simulink model "Drone_BBall_Friendly"  (R2020a)
settings: Solver=FixedStepAuto  StartTime=0.0  StopTime=60  FixedStep=.001  RelTol=1e-3
values from neighbouring files (symbols this model uses):
  b = .25*m    (= 0.25)    [Run_Match.m]
  b_ball = .02*m_ball    (= 0.01)    [Run_Match.m]
  b_F_hook = 100    [Run_Match.m]
  b_F_hoop = m_ball * 50    (= 25)    [Run_Match.m]
  b_F_R = m * 20    (= 20)    [Run_Match.m]
  b_F_R_ball = m_ball * 10    (= 5)    [Run_Match.m]
  b_F_R_hook = m_hook * 100    (= 10)    [Run_Match.m]
  B_hook = r_hook^2*6*m_ball*g    (= 0.2943)    [Run_Match.m]
  b_hook = 0.05*m_hook    (= 0.005)    [Run_Match.m]
  b_tether = 1    [Run_Match.m]
  b_th = .1*J    (= 0.0192708333333)    [Run_Match.m]
  b_th_ball = .05*J_ball    (= 0.0009)    [Run_Match.m]
  b_x_net = 80*m_ball*g    (= 392.4)    [Run_Match.m]
  b_y_net = .4*m_ball*g    (= 1.962)    [Run_Match.m]
  drone = struct([])    [Run_Match.m]    (also in animate_drone_bball.m = [-r+w -r-w -r -r r r r+w r-w;             h    h  h  0 0 h  )
  g = 9.81    [Run_Match.m]
  J = 1/4*m*r^2 + 1/12*m*(2*(r+r_M_R))^2    (= 0.192708333333)    [Run_Match.m]
  J_ball = 2/5*m_ball*r_ball^2    (= 0.018)    [Run_Match.m]
  k_f = 4    [Run_Match.m]
  k_F_hook = 10000    [Run_Match.m]
  k_F_hoop = m_ball * 5000    (= 2500)    [Run_Match.m]
  k_F_R = m * 10000    (= 10000)    [Run_Match.m]
  k_F_R_ball = m_ball * 10000    (= 5000)    [Run_Match.m]
  k_F_R_hook = m_hook * 10000    (= 1000)    [Run_Match.m]
  k_tether = 40    [Run_Match.m]
  k_x_net = 200*m_ball*g    (= 981)    [Run_Match.m]
  k_y_net = .5*m_ball*g    (= 2.4525)    [Run_Match.m]
  L_tether = 1.0    (= 1)    [Run_Match.m]
  m = 1    [Run_Match.m]
  m_ball = .5    (= 0.5)    [Run_Match.m]
  m_hook = 0.1*m    (= 0.1)    [Run_Match.m]
  mu_f = .2    (= 0.2)    [Run_Match.m]
  mu_f_gnd = 0.5    [Run_Match.m]
  p_ball_0 = [0; r_ball]    [Run_Match.m]
  p_ball_dot_0 = [0; 12]    [Run_Match.m]
  p_emp = [0; -.4]    [Run_Match.m]
  p_emp_dot = [0; -5]    [Run_Match.m]
  p_hoop = [7.5 8; 8.5 8; -8.5 8; -7.5 8]'    [Run_Match.m]
  p_tether = [0; -0.259]    [Run_Match.m]
  r = 0.5    [Run_Match.m]    (also in animate_drone_bball.m = 0.475)
  r_ball = .3    (= 0.3)    [Run_Match.m]
  r_hook = 0.1    [Run_Match.m]
  r_M_R = 0.25*r    (= 0.125)    [Run_Match.m]
  T_0 = m*g    (= 9.81)    [Run_Match.m]
  T_max = 4*m*g    (= 39.24)    [Run_Match.m]
  T_tau = 0.1    [Run_Match.m]
undefined symbols (not defined in the file or in its folder): clock
libraries: dspswit3 x22, simulink x10, dspmathops x2
(part 3 of 3)

== system Drone_BBall_Friendly/Drone 1 Dynamics/Quadcopter Plant/Rotational Dynamics ==
  M : Inport
  Fcn1 : Fcn  Expr=u*abs(u)
  Gain : Gain  Gain=b_th
  Gain1 : Gain  Gain=1/J
  Integrator : Integrator  InitialCondition=param.X_0(6)
  Integrator1 : Integrator  InitialCondition=param.X_0(5)
  Sum2 : Sum  Inputs=|+-
  Wrap Angle : Subsystem
  theta : Outport  VectorParamsAs1DForOutWhenUnconnected=off
  theta_dot : Outport  Port=2  VectorParamsAs1DForOutWhenUnconnected=off
  wires:
  Integrator1/1 -> Wrap Angle/1(raw)
  Integrator/1 -> Integrator1/1, Fcn1/1, theta_dot/1
  Gain1/1 -> Integrator/1
  Wrap Angle/1(wrap) -> theta/1
  Fcn1/1 -> Gain/1
  M/1 -> Sum2/1
  Gain/1 -> Sum2/2
  Sum2/1 -> Gain1/1

== system Drone_BBall_Friendly/Drone 1 Dynamics/Quadcopter Plant/Thrust Dynamics ==
  T_d : Inport
  Gain : Gain  Gain=1/T_tau
  Integrator : Integrator  InitialCondition=T_0/2
  Sum : Sum  Inputs=|+-
  Thrust Limit : Saturate  UpperLimit=T_max  LowerLimit=0
  T : Outport  VectorParamsAs1DForOutWhenUnconnected=off
  wires:
  Gain/1 -> Integrator/1
  Sum/1 -> Gain/1
  Thrust Limit/1 -> Sum/1
  T_d/1 -> Thrust Limit/1
  Integrator/1 -> T/1, Sum/2

== system Drone_BBall_Friendly/Drone 1 Dynamics/Quadcopter Plant/Thrust Dynamics L ==
  T_d : Inport
  Gain : Gain  Gain=1/T_tau
  Integrator : Integrator  InitialCondition=T_0/2
  Sum : Sum  Inputs=|+-
  Thrust Limit : Saturate  UpperLimit=T_max  LowerLimit=0
  T : Outport  VectorParamsAs1DForOutWhenUnconnected=off
  wires:
  Gain/1 -> Integrator/1
  Sum/1 -> Gain/1
  Thrust Limit/1 -> Sum/1
  T_d/1 -> Thrust Limit/1
  Integrator/1 -> T/1, Sum/2

== system Drone_BBall_Friendly/Drone 1 Dynamics/Quadcopter Plant/Thrust Resultants ==
  T_L : Inport
  T_R : Inport  Port=2
  Theta : Inport  Port=3
  Gain : Gain  Gain=r
  Mux : Mux  Inputs=3
  Product : Product
  Product1 : Product
  Sin : Trigonometry
  Sin1 : Trigonometry  Operator=cos
  Sum : Sum  Inputs=|++
  Sum1 : Sum  Inputs=+-|
  "FM " : Outport  VectorParamsAs1DForOutWhenUnconnected=off
  wires:
  T_L/1 -> Sum/1, Sum1/1
  T_R/1 -> Sum/2, Sum1/2
  Gain/1 -> Mux/3  "M"
  Sum1/1 -> Gain/1
  Sum/1 -> Product1/1, Product/1
  Sin1/1 -> Product1/2
  Theta/1 -> Sin/1, Sin1/1
  Product/1 -> Mux/1  "F_x"
  Sin/1 -> Product/2
  Mux/1 -> "FM "/1
  Product1/1 -> Mux/2  "F_y"

== system Drone_BBall_Friendly/Drone 2 Dynamics/Hook Plant/Ground Reactions ==
  X : Inport
  Constant1 : Constant  Value=0
  Demux : Demux  Outputs=6
  Gain : Gain  Gain=-k_F_R_hook
  Gain4 : Gain  Gain=-b_F_R_hook
  Gain6 : Gain  Gain=-k_f
  Less Than1 : RelationalOperator  Operator=>  OutDataTypeStr=boolean  RndMeth=Simplest
  Mux : Mux  Inputs=2
  Product2 : Product
  Product5 : Product  Inputs=3
  Saturation : Saturate  UpperLimit=Inf  LowerLimit=0
  Saturation1 : Saturate  UpperLimit=mu_f  LowerLimit=-mu_f
  Sum1 : Sum  Inputs=|++
  Terminator : Terminator
  Terminator1 : Terminator
  Terminator2 : Terminator
  F_R : Outport  VectorParamsAs1DForOutWhenUnconnected=off
  wires:
  Gain6/1 -> Saturation1/1
  Saturation1/1 -> Product5/1
  Saturation/1 -> Product2/2, Product5/2
  Demux/1 -> Terminator/1
  Mux/1 -> F_R/1
  Product2/1 -> Mux/2
  Demux/5 -> Terminator1/1
  Constant1/1 -> Less Than1/1
  Demux/3 -> Gain/1, Less Than1/2
  Product5/1 -> Mux/1
  Gain4/1 -> Sum1/2
  Less Than1/1 -> Product5/3, Product2/1
  Sum1/1 -> Saturation/1
  Demux/2 -> Gain6/1
  Demux/4 -> Gain4/1
  Gain/1 -> Sum1/1
  X/1 -> Demux/1
  Demux/6 -> Terminator2/1

== system Drone_BBall_Friendly/Drone 2 Dynamics/Hook Plant/Hook Dynamics ==
  X_hook : Inport
  X_ball : Inport  Port=2
  mag_on : Inport  Port=3
  Constant : Constant  Value=0
  Constant1 : Constant  Value=r_ball
  Constant2 : Constant  Value=r_ball
  Constant3 : Constant  Value=r_hook
  Divide1 : Product  Inputs=**/
  Divide2 : Product  Inputs=*/
  Dot Product : DotProduct  InputSameDT=on  OutDataTypeStr=Inherit: Inherit via internal rule
  Dot Product1 : DotProduct  InputSameDT=on  OutDataTypeStr=Inherit: Inherit via internal rule
  Gain : Gain  Gain=r_ball
  Gain1 : Gain  Gain=-k_f
  Gain2 : Gain  Gain=b_F_hook
  Gain3 : Gain  Gain=k_F_hook
  Gain6 : Gain  Gain=B_hook
  Gain7 : Gain  Gain=[0 1;-1 0]  Multiplication=Matrix(K*u)
  GreaterThan : RelationalOperator  Operator=>  OutDataTypeStr=boolean  RndMeth=Simplest
  Norm : Fcn  Expr=sqrt(u(1)^2+u(2)^2)+1e-10
  Product : Product  Inputs=3
  Product{1..5} (5 alike) : Product
  Saturation : Saturate  UpperLimit=0  LowerLimit=-Inf
  Saturation1 : Saturate  UpperLimit=mu_f  LowerLimit=-mu_f
  Selector : Selector  InputPortWidth=6  IndexOptions=Index vector (dialog)  Indices=[1 3]  OutputSizes=1
  Selector1 : Selector  InputPortWidth=6  IndexOptions=Index vector (dialog)  Indices=[6]  OutputSizes=1
  Selector2 : Selector  InputPortWidth=6  IndexOptions=Index vector (dialog)  Indices=[2 4]  OutputSizes=1
  Square : Math  Operator=square  SignedPower=on  SaturateOnIntegerOverflow=on
  Sum : Sum  Inputs=+-
  Sum1 : Sum  Inputs=+||+|||+
  Sum2 : Sum  Inputs=+|+
  Sum3 : Sum  Inputs=-|+
  Sum4 : Sum  Inputs=++|
  Sum5 : Sum  Inputs=+-+
  F_ball : Outport  VectorParamsAs1DForOutWhenUnconnected=off
  M_ball : Outport  Port=2  VectorParamsAs1DForOutWhenUnconnected=off
  wires:
  Gain/1 -> M_ball/1
  mag_on/1 -> Divide1/2
  X_hook/1 -> Sum/1
  X_ball/1 -> Sum/2
  Sum/1 -> Selector1/1, Selector2/1, Selector/1
  Selector/1 -> Divide2/1, Norm/1
  Sum3/1 -> Product1/2, GreaterThan/2  "Overlap Distance"
  Constant/1 -> GreaterThan/1
  GreaterThan/1 -> Product1/1, Product3/2
  Product3/1 -> Gain2/1
  Sum1/1 -> F_ball/1
  Dot Product1/1 -> Gain1/1
  Gain2/1 -> Sum2/1
  Gain3/1 -> Sum2/2
  Product5/1 -> Product2/1, Gain/1
  Divide1/1 -> Gain6/1
  Gain6/1 -> Sum1/3  "Magnetic Force"
  Norm/1 -> Sum5/1, Divide2/2, Product/2, Sum3/2  "radius"
  Constant1/1 -> Sum3/1
  Divide2/1 -> Divide1/1, Product4/2, Gain7/1, Dot Product/2  "Normalized Pos Vector"
  Dot Product/1 -> Product3/1
  Product1/1 -> Gain3/1
  Square/1 -> Divide1/3  "Squared Distance"
  Gain7/1 -> Product/3, Product2/2, Dot Product1/2  "Tangent Vector"
  Product/1 -> Sum4/2
  Selector2/1 -> Sum4/1
  Sum4/1 -> Dot Product/1, Dot Product1/1
  Selector1/1 -> Product/1  "theta_dot"
  Gain1/1 -> Saturation1/1
  Product4/1 -> Sum1/2  "Normal Force"
  Product2/1 -> Sum1/1  "Friction Force"
  Saturation/1 -> Product5/2, Product4/1
  Sum2/1 -> Saturation/1
  Saturation1/1 -> Product5/1
  Constant2/1 -> Sum5/2
  Constant3/1 -> Sum5/3
  Sum5/1 -> Square/1  "Magnet Distance"

== system Drone_BBall_Friendly/Drone 2 Dynamics/Hook Plant/Linear Dynamics ==
  F : Inport
  Gain : Gain  Gain=1/m_hook
  Gain1 : Gain  Gain=b_hook
  Integrator : Integrator  InitialCondition=param.X_0([1 3])+p_tether+[0;-L_tether]
  Integrator1 : Integrator  InitialCondition=param.X_0([2 4])
  Norm : Fcn  Expr=sqrt(u(1)^2+u(2)^2)
  Product : Product
  Sum3 : Sum  Inputs=+-
  p : Outport  VectorParamsAs1DForOutWhenUnconnected=off
  p_dot : Outport  Port=2  VectorParamsAs1DForOutWhenUnconnected=off
  wires:
  Gain1/1 -> Sum3/2
  Integrator1/1 -> Integrator/1, Norm/1, Product/1, p_dot/1
  Norm/1 -> Product/2
  Product/1 -> Gain1/1
  F/1 -> Sum3/1
  Sum3/1 -> Gain/1
  Gain/1 -> Integrator1/1
  Integrator/1 -> p/1

== system Drone_BBall_Friendly/Drone 2 Dynamics/Hook Plant/Tether Dynamics ==
  note: theta_hook = 0
      | (point particle)
  X_drone : Inport
  X_hook : Inport  Port=2
  Constant1 : Constant  Value=0
  Constant2 : Constant  Value=L_tether
  Constant5 : Constant  Value=p_tether
  Divide1 : Product  Inputs=*/
  Dot Product{,3..5} (4 alike) : DotProduct  InputSameDT=on  OutDataTypeStr=Inherit: Inherit via internal rule
  Gain : Gain  Gain=-1
  Gain2 : Gain  Gain=[0 1;-1 0]  Multiplication=Matrix(K*u)
  Gain3 : Gain  Gain=b_tether
  Gain5 : Gain  Gain=k_tether
  Gain8 : Gain  Gain=[0 1;-1 0]  Multiplication=Matrix(K*u)
  GreaterThan1 : RelationalOperator  Operator=>  OutDataTypeStr=boolean  RndMeth=Simplest
  Multiply1 : Product
  Mux2 : Mux  Inputs=2
  Norm1 : Fcn  Expr=sqrt(u(1)^2+u(2)^2)+1e-10
  Normalization : dspmathops/Normalization  NormType=2-norm  Bias=1e-10  NormOver=Each column  Dimension=1  roundingMode=Floor  overflowMode=off  accumDataTypeStr=Inherit: Same as product output  accumLastDataTypeStr=Inherit: Same as product output  outputDataTypeStr=Inherit: Same as product output  outputMin=[]  outputMax=[]  outputLastDataTypeStr=Inherit: Same as product output
  Product2 : Product
  Product6 : Product
  Rotation Matrix CW : Subsystem
  Saturation : Saturate  UpperLimit=Inf  LowerLimit=0
  Selector1 : Selector  InputPortWidth=6  IndexOptions=Index vector (dialog)  Indices=[1 3]  OutputSizes=1
  Selector2 : Selector  InputPortWidth=6  IndexOptions=Index vector (dialog)  Indices=[5]  OutputSizes=1
  Selector3 : Selector  InputPortWidth=6  IndexOptions=Index vector (dialog)  Indices=[2 4]  OutputSizes=1
  Selector5 : Selector  InputPortWidth=6  IndexOptions=Index vector (dialog)  Indices=[6]  OutputSizes=1
  Sum : Sum  Inputs=+|-
  Sum11 : Sum
  Sum3 : Sum  Inputs=+|+
  Sum4 : Sum  Inputs=-+
  Sum8 : Sum  Inputs=+|||+
  F_tether : Outport  VectorParamsAs1DForOutWhenUnconnected=off
  M_tether : Outport  Port=2  VectorParamsAs1DForOutWhenUnconnected=off
  F_tether_r : Outport  Port=3  VectorParamsAs1DForOutWhenUnconnected=off
  wires:
  Constant1/1 -> GreaterThan1/2
  Sum11/1 -> Norm1/1, Divide1/1
  Sum4/1 -> Gain5/1, GreaterThan1/1  "Overlap Distance"
  X_drone/1 -> Sum/1
  Dot Product/1 -> Gain3/1
  Selector2/1 -> Rotation Matrix CW/2(theta)
  X_hook/1 -> Sum/2
  Gain5/1 -> Sum3/2
  Saturation/1 -> Product2/1
  Divide1/1 -> Product6/2, Dot Product/2  "Normalized Hook Pos"
  Norm1/1 -> Sum4/2, Divide1/2  "distance"
  Sum8/1 -> Dot Product/1
  GreaterThan1/1 -> Product2/2
  Gain3/1 -> Sum3/1
  Sum3/1 -> Saturation/1
  Selector5/1 -> Multiply1/2
  Product2/1 -> Product6/1
  Constant2/1 -> Sum4/1
  Sum/1 -> Selector1/1, Selector2/1, Selector5/1, Selector3/1
  Constant5/1 -> Rotation Matrix CW/1(p)
  Rotation Matrix CW/1(R(theta)*p) -> Normalization/1, Sum11/1, Gain8/1
  Gain8/1 -> Dot Product3/1, Multiply1/1
  Multiply1/1 -> Sum8/1
  Selector3/1 -> Sum8/2
  Selector1/1 -> Sum11/2
  Dot Product3/1 -> M_tether/1
  Product6/1 -> F_tether/1, Dot Product5/2, Dot Product4/2, Dot Product3/2
  Normalization/1 -> Gain/1  "Normalized Tether Pos"
  Gain2/1 -> Dot Product5/1
  Dot Product5/1 -> Mux2/1
  Dot Product4/1 -> Mux2/2
  Mux2/1 -> F_tether_r/1
  Gain/1 -> Gain2/1, Dot Product4/1

== system Drone_BBall_Friendly/Drone 2 Dynamics/Quadcopter Plant/Ceiling Reactions ==
  X : Inport
  Constant1 : Constant  Value=0
  Constant2 : Constant  Value=16-r
  Demux : Demux  Outputs=6
  Gain1 : Gain  Gain=r_M_R
  Gain10 : Gain  Gain=-k_f
  Gain12 : Gain  Gain=2
  Gain13 : Gain  Gain=r_M_R
  Gain4 : Gain  Gain=-b_F_R
  Gain6 : Gain  Gain=-k_F_R
  Gain8 : Gain  Gain=r
  Gain9 : Gain  Gain=r
  Less Than1 : RelationalOperator  Operator=<  OutDataTypeStr=boolean  RndMeth=Simplest
  Mux : Mux  Inputs=3
  Product5 : Product
  Product6 : Product  Inputs=3
  Product7 : Product
  Saturation : Saturate  UpperLimit=0  LowerLimit=-Inf
  Saturation1 : Saturate  UpperLimit=mu_f_gnd  LowerLimit=-mu_f_gnd
  Sin1 : Trigonometry
  Sin2 : Trigonometry  Operator=cos
  Sum3 : Sum  Inputs=|++
  Sum4 : Sum  Inputs=+-+
  Sum5 : Sum  Inputs=--|
  Sum6 : Sum  Inputs=++|
  Terminator : Terminator
  FM_R : Outport  VectorParamsAs1DForOutWhenUnconnected=off
  wires:
  Demux/2 -> Sum5/1
  Gain10/1 -> Saturation1/1
  Saturation1/1 -> Product6/1
  Saturation/1 -> Product5/2, Product6/2
  Demux/1 -> Terminator/1
  Product5/1 -> Product7/1, Mux/2
  Constant1/1 -> Less Than1/1
  Sum4/1 -> Less Than1/2, Gain6/1
  Demux/3 -> Sum4/3
  Product6/1 -> Mux/1, Gain8/1
  Demux/6 -> Gain9/1
  Gain4/1 -> Sum3/2
  Less Than1/1 -> Product6/3, Product5/1
  Sum3/1 -> Saturation/1
  Gain9/1 -> Sum5/2
  Sum5/1 -> Gain10/1
  Demux/4 -> Gain4/1
  Gain6/1 -> Sum3/1
  X/1 -> Demux/1
  Demux/5 -> Gain12/1
  Gain12/1 -> Sin2/1, Sin1/1
  Sin1/1 -> Gain13/1
  Gain13/1 -> Product7/2  "Moment arm of normal reaction force"
  Gain8/1 -> Sum6/1
  Sum6/1 -> Mux/3
  Product7/1 -> Sum6/2
  Mux/1 -> FM_R/1
  Sin2/1 -> Gain1/1
  Constant2/1 -> Sum4/2
  Gain1/1 -> Sum4/1

== system Drone_BBall_Friendly/Drone 2 Dynamics/Quadcopter Plant/Ground Reactions ==
  X : Inport
  Constant1 : Constant  Value=0
  Constant2 : Constant  Value=r
  Demux : Demux  Outputs=6
  Gain1 : Gain  Gain=r_M_R
  Gain10 : Gain  Gain=-k_f
  Gain12 : Gain  Gain=2
  Gain13 : Gain  Gain=r_M_R
  Gain4 : Gain  Gain=-b_F_R
  Gain6 : Gain  Gain=-k_F_R
  Gain8 : Gain  Gain=-r
  Gain9 : Gain  Gain=r
  Less Than1 : RelationalOperator  Operator=>  OutDataTypeStr=boolean  RndMeth=Simplest
  Mux : Mux  Inputs=3
  Product5 : Product
  Product6 : Product  Inputs=3
  Product7 : Product
  Saturation : Saturate  UpperLimit=Inf  LowerLimit=0
  Saturation1 : Saturate  UpperLimit=mu_f_gnd  LowerLimit=-mu_f_gnd
  Sin1 : Trigonometry
  Sin2 : Trigonometry  Operator=cos
  Sum3 : Sum  Inputs=|++
  Sum4 : Sum  Inputs=+-+
  Sum5 : Sum  Inputs=+-|
  Sum6 : Sum  Inputs=+-|
  Terminator : Terminator
  FM_R : Outport  VectorParamsAs1DForOutWhenUnconnected=off
  wires:
  Demux/2 -> Sum5/1
  Gain10/1 -> Saturation1/1
  Saturation1/1 -> Product6/1
  Saturation/1 -> Product5/2, Product6/2
  Demux/1 -> Terminator/1
  Product5/1 -> Product7/1, Mux/2
  Constant1/1 -> Less Than1/1
  Sum4/1 -> Less Than1/2, Gain6/1
  Demux/3 -> Sum4/3
  Product6/1 -> Gain8/1, Mux/1
  Demux/6 -> Gain9/1
  Gain4/1 -> Sum3/2
  Less Than1/1 -> Product6/3, Product5/1
  Sum3/1 -> Saturation/1
  Gain9/1 -> Sum5/2
  Sum5/1 -> Gain10/1
  Demux/4 -> Gain4/1
  Gain6/1 -> Sum3/1
  X/1 -> Demux/1
  Demux/5 -> Gain12/1
  Gain12/1 -> Sin2/1, Sin1/1
  Sin1/1 -> Gain13/1
  Gain13/1 -> Product7/2  "Moment arm of normal reaction force"
  Gain8/1 -> Sum6/1
  Sum6/1 -> Mux/3
  Product7/1 -> Sum6/2
  Mux/1 -> FM_R/1
  Sin2/1 -> Gain1/1
  Constant2/1 -> Sum4/2
  Gain1/1 -> Sum4/1

== system Drone_BBall_Friendly/Drone 2 Dynamics/Quadcopter Plant/Left Wall Reactions ==
  X : Inport
  Constant1 : Constant  Value=0
  Constant2 : Constant  Value=r-12
  Demux : Demux  Outputs=6
  Gain1 : Gain  Gain=r_M_R
  Gain10 : Gain  Gain=-k_f
  Gain12 : Gain  Gain=2
  Gain13 : Gain  Gain=r_M_R
  Gain4 : Gain  Gain=-b_F_R
  Gain6 : Gain  Gain=-k_F_R
  Gain8 : Gain  Gain=r
  Gain9 : Gain  Gain=r
  Less Than1 : RelationalOperator  Operator=<  OutDataTypeStr=boolean  RndMeth=Simplest
  Mux : Mux  Inputs=3
  Product5 : Product
  Product6 : Product  Inputs=3
  Product7 : Product
  Saturation : Saturate  UpperLimit=Inf  LowerLimit=0
  Saturation1 : Saturate  UpperLimit=mu_f_gnd  LowerLimit=-mu_f_gnd
  Sin1 : Trigonometry
  Sin2 : Trigonometry  Operator=cos
  Sum3 : Sum  Inputs=|++
  Sum4 : Sum  Inputs=--+
  Sum5 : Sum  Inputs=|++
  Sum6 : Sum  Inputs=++|
  Terminator : Terminator
  FM_R : Outport  VectorParamsAs1DForOutWhenUnconnected=off
  wires:
  Demux/4 -> Sum5/1
  Gain10/1 -> Saturation1/1
  Saturation1/1 -> Product6/3
  Saturation/1 -> Product5/1, Product6/2
  Product5/1 -> Product7/1, Mux/1
  Constant1/1 -> Less Than1/2
  Sum4/1 -> Less Than1/1, Gain6/1
  Demux/1 -> Sum4/3
  Product6/1 -> Mux/2, Gain8/1
  Demux/6 -> Gain9/1
  Gain4/1 -> Sum3/2
  Less Than1/1 -> Product5/2, Product6/1
  Sum3/1 -> Saturation/1
  Gain9/1 -> Sum5/2
  Sum5/1 -> Gain10/1
  Demux/2 -> Gain4/1
  Gain6/1 -> Sum3/1
  X/1 -> Demux/1
  Demux/5 -> Gain12/1
  Gain12/1 -> Sin2/1, Sin1/1
  Sin1/1 -> Gain13/1
  Gain13/1 -> Product7/2  "Moment arm of normal reaction force"
  Gain8/1 -> Sum6/1
  Sum6/1 -> Mux/3
  Product7/1 -> Sum6/2
  Mux/1 -> FM_R/1
  Sin2/1 -> Gain1/1
  Constant2/1 -> Sum4/2
  Gain1/1 -> Sum4/1
  Demux/3 -> Terminator/1

== system Drone_BBall_Friendly/Drone 2 Dynamics/Quadcopter Plant/Linear Dynamics ==
  F : Inport
  Gain2 : Gain  Gain=1/m
  Gain5 : Gain  Gain=b
  Integrator4 : Integrator  InitialCondition=param.X_0([2 4])
  Integrator5 : Integrator  InitialCondition=param.X_0([1 3])
  Norm : Fcn  Expr=sqrt(u(1)^2+u(2)^2)
  Product4 : Product
  Sum3 : Sum  Inputs=+-
  p : Outport  VectorParamsAs1DForOutWhenUnconnected=off
  p_dot : Outport  Port=2  VectorParamsAs1DForOutWhenUnconnected=off
  wires:
  Integrator5/1 -> p/1
  F/1 -> Sum3/1
  Norm/1 -> Product4/2
  Integrator4/1 -> Integrator5/1, Norm/1, Product4/1, p_dot/1
  Sum3/1 -> Gain2/1
  Gain2/1 -> Integrator4/1
  Gain5/1 -> Sum3/2
  Product4/1 -> Gain5/1

== system Drone_BBall_Friendly/Drone 2 Dynamics/Quadcopter Plant/Right Wall Reactions ==
  X : Inport
  Constant1 : Constant  Value=0
  Constant2 : Constant  Value=12-r
  Demux : Demux  Outputs=6
  Gain1 : Gain  Gain=r_M_R
  Gain10 : Gain  Gain=-k_f
  Gain12 : Gain  Gain=2
  Gain13 : Gain  Gain=r_M_R
  Gain4 : Gain  Gain=-b_F_R
  Gain6 : Gain  Gain=-k_F_R
  Gain8 : Gain  Gain=r
  Gain9 : Gain  Gain=r
  Less Than1 : RelationalOperator  Operator=>  OutDataTypeStr=boolean  RndMeth=Simplest
  Mux : Mux  Inputs=3
  Product5 : Product
  Product6 : Product  Inputs=3
  Product7 : Product
  Saturation : Saturate  UpperLimit=0  LowerLimit=-Inf
  Saturation1 : Saturate  UpperLimit=mu_f_gnd  LowerLimit=-mu_f_gnd
  Sin1 : Trigonometry
  Sin2 : Trigonometry  Operator=cos
  Sum3 : Sum  Inputs=|++
  Sum4 : Sum  Inputs=--+
  Sum5 : Sum  Inputs=|-+
  Sum6 : Sum  Inputs=+-|
  Terminator : Terminator
  FM_R : Outport  VectorParamsAs1DForOutWhenUnconnected=off
  wires:
  Demux/4 -> Sum5/1
  Gain10/1 -> Saturation1/1
  Saturation1/1 -> Product6/3
  Saturation/1 -> Product5/1, Product6/2
  Product5/1 -> Product7/1, Mux/1
  Constant1/1 -> Less Than1/2
  Sum4/1 -> Less Than1/1, Gain6/1
  Demux/1 -> Sum4/3
  Product6/1 -> Mux/2, Gain8/1
  Demux/6 -> Gain9/1
  Gain4/1 -> Sum3/2
  Less Than1/1 -> Product5/2, Product6/1
  Sum3/1 -> Saturation/1
  Gain9/1 -> Sum5/2
  Sum5/1 -> Gain10/1
  Demux/2 -> Gain4/1
  Gain6/1 -> Sum3/1
  X/1 -> Demux/1
  Demux/5 -> Gain12/1
  Gain12/1 -> Sin2/1, Sin1/1
  Sin1/1 -> Gain13/1
  Gain13/1 -> Product7/2  "Moment arm of normal reaction force"
  Gain8/1 -> Sum6/1
  Sum6/1 -> Mux/3
  Product7/1 -> Sum6/2
  Mux/1 -> FM_R/1
  Sin2/1 -> Gain1/1
  Constant2/1 -> Sum4/2
  Gain1/1 -> Sum4/1
  Demux/3 -> Terminator/1

== system Drone_BBall_Friendly/Drone 2 Dynamics/Quadcopter Plant/Rotational Dynamics ==
  M : Inport
  Fcn1 : Fcn  Expr=u*abs(u)
  Gain : Gain  Gain=b_th
  Gain1 : Gain  Gain=1/J
  Integrator : Integrator  InitialCondition=param.X_0(6)
  Integrator1 : Integrator  InitialCondition=param.X_0(5)
  Sum2 : Sum  Inputs=|+-
  Wrap Angle : Subsystem
  theta : Outport  VectorParamsAs1DForOutWhenUnconnected=off
  theta_dot : Outport  Port=2  VectorParamsAs1DForOutWhenUnconnected=off
  wires:
  Integrator1/1 -> Wrap Angle/1(raw)
  Integrator/1 -> Integrator1/1, Fcn1/1, theta_dot/1
  Gain1/1 -> Integrator/1
  Wrap Angle/1(wrap) -> theta/1
  Fcn1/1 -> Gain/1
  M/1 -> Sum2/1
  Gain/1 -> Sum2/2
  Sum2/1 -> Gain1/1

== system Drone_BBall_Friendly/Drone 2 Dynamics/Quadcopter Plant/Thrust Dynamics ==
  T_d : Inport
  Gain : Gain  Gain=1/T_tau
  Integrator : Integrator  InitialCondition=T_0/2
  Sum : Sum  Inputs=|+-
  Thrust Limit : Saturate  UpperLimit=T_max  LowerLimit=0
  T : Outport  VectorParamsAs1DForOutWhenUnconnected=off
  wires:
  Gain/1 -> Integrator/1
  Sum/1 -> Gain/1
  Thrust Limit/1 -> Sum/1
  T_d/1 -> Thrust Limit/1
  Integrator/1 -> T/1, Sum/2

== system Drone_BBall_Friendly/Drone 2 Dynamics/Quadcopter Plant/Thrust Dynamics L ==
  T_d : Inport
  Gain : Gain  Gain=1/T_tau
  Integrator : Integrator  InitialCondition=T_0/2
  Sum : Sum  Inputs=|+-
  Thrust Limit : Saturate  UpperLimit=T_max  LowerLimit=0
  T : Outport  VectorParamsAs1DForOutWhenUnconnected=off
  wires:
  Gain/1 -> Integrator/1
  Sum/1 -> Gain/1
  Thrust Limit/1 -> Sum/1
  T_d/1 -> Thrust Limit/1
  Integrator/1 -> T/1, Sum/2

== system Drone_BBall_Friendly/Drone 2 Dynamics/Quadcopter Plant/Thrust Resultants ==
  T_L : Inport
  T_R : Inport  Port=2
  Theta : Inport  Port=3
  Gain : Gain  Gain=r
  Mux : Mux  Inputs=3
  Product : Product
  Product1 : Product
  Sin : Trigonometry
  Sin1 : Trigonometry  Operator=cos
  Sum : Sum  Inputs=|++
  Sum1 : Sum  Inputs=+-|
  "FM " : Outport  VectorParamsAs1DForOutWhenUnconnected=off
  wires:
  T_L/1 -> Sum/1, Sum1/1
  T_R/1 -> Sum/2, Sum1/2
  Gain/1 -> Mux/3  "M"
  Sum1/1 -> Gain/1
  Product1/1 -> Mux/2  "F_y"
  Sin1/1 -> Product1/2
  Theta/1 -> Sin/1, Sin1/1
  Product/1 -> Mux/1  "F_x"
  Sin/1 -> Product/2
  Sum/1 -> Product1/1, Product/1
  Mux/1 -> "FM "/1

== system Drone_BBall_Friendly/EMP Mechanics//Dynamics/EMP Dynamics 1/Rotation Matrx ==
  p : Inport
  theta : Inport  Port=2
  Cos : Trigonometry  Operator=cos
  Demux : Demux  Outputs=2
  Demux1 : Demux  Outputs=2
  Mux3 : Mux  Inputs=2
  Product : Product
  Product1 : Product
  Sin : Trigonometry
  Sum1 : Sum
  Sum2 : Sum  Inputs=+-
  R(theta)*p : Outport  VectorParamsAs1DForOutWhenUnconnected=off
  wires:
  p/1 -> Product/2, Product1/2
  Sum2/1 -> Mux3/2
  Sin/1 -> Product1/1
  theta/1 -> Cos/1, Sin/1
  Cos/1 -> Product/1
  Sum1/1 -> Mux3/1
  Mux3/1 -> R(theta)*p/1
  Product/1 -> Demux/1
  Product1/1 -> Demux1/1
  Demux/1 -> Sum1/1
  Demux1/2 -> Sum1/2
  Demux1/1 -> Sum2/2
  Demux/2 -> Sum2/1

== system Drone_BBall_Friendly/EMP Mechanics//Dynamics/EMP Dynamics 1/Rotation Matrx1 ==
  p : Inport
  theta : Inport  Port=2
  Cos : Trigonometry  Operator=cos
  Demux : Demux  Outputs=2
  Demux1 : Demux  Outputs=2
  Mux3 : Mux  Inputs=2
  Product : Product
  Product1 : Product
  Sin : Trigonometry
  Sum1 : Sum
  Sum2 : Sum  Inputs=+-
  R(theta)*p : Outport  VectorParamsAs1DForOutWhenUnconnected=off
  wires:
  p/1 -> Product/2, Product1/2
  Sum2/1 -> Mux3/2
  Sin/1 -> Product1/1
  theta/1 -> Cos/1, Sin/1
  Cos/1 -> Product/1
  Sum1/1 -> Mux3/1
  Mux3/1 -> R(theta)*p/1
  Product/1 -> Demux/1
  Product1/1 -> Demux1/1
  Demux/1 -> Sum1/1
  Demux1/2 -> Sum1/2
  Demux1/1 -> Sum2/2
  Demux/2 -> Sum2/1

== system Drone_BBall_Friendly/EMP Mechanics//Dynamics/EMP Dynamics 2/Rotation Matrx ==
  p : Inport
  theta : Inport  Port=2
  Cos : Trigonometry  Operator=cos
  Demux : Demux  Outputs=2
  Demux1 : Demux  Outputs=2
  Mux3 : Mux  Inputs=2
  Product : Product
  Product1 : Product
  Sin : Trigonometry
  Sum1 : Sum
  Sum2 : Sum  Inputs=+-
  R(theta)*p : Outport  VectorParamsAs1DForOutWhenUnconnected=off
  wires:
  p/1 -> Product/2, Product1/2
  Sum2/1 -> Mux3/2
  Sin/1 -> Product1/1
  theta/1 -> Cos/1, Sin/1
  Cos/1 -> Product/1
  Sum1/1 -> Mux3/1
  Mux3/1 -> R(theta)*p/1
  Product/1 -> Demux/1
  Product1/1 -> Demux1/1
  Demux/1 -> Sum1/1
  Demux1/2 -> Sum1/2
  Demux1/1 -> Sum2/2
  Demux/2 -> Sum2/1

== system Drone_BBall_Friendly/EMP Mechanics//Dynamics/EMP Dynamics 2/Rotation Matrx1 ==
  p : Inport
  theta : Inport  Port=2
  Cos : Trigonometry  Operator=cos
  Demux : Demux  Outputs=2
  Demux1 : Demux  Outputs=2
  Mux3 : Mux  Inputs=2
  Product : Product
  Product1 : Product
  Sin : Trigonometry
  Sum1 : Sum
  Sum2 : Sum  Inputs=+-
  R(theta)*p : Outport  VectorParamsAs1DForOutWhenUnconnected=off
  wires:
  p/1 -> Product/2, Product1/2
  Sum2/1 -> Mux3/2
  Sin/1 -> Product1/1
  theta/1 -> Cos/1, Sin/1
  Cos/1 -> Product/1
  Sum1/1 -> Mux3/1
  Mux3/1 -> R(theta)*p/1
  Product/1 -> Demux/1
  Product1/1 -> Demux1/1
  Demux/1 -> Sum1/1
  Demux1/2 -> Sum1/2
  Demux1/1 -> Sum2/2
  Demux/2 -> Sum2/1

== system Drone_BBall_Friendly/Drone 1 Dynamics/Hook Plant/Tether Dynamics/Rotation Matrix CW ==
  p : Inport
  theta : Inport  Port=2
  Cos : Trigonometry  Operator=cos
  Demux : Demux  Outputs=2
  Demux1 : Demux  Outputs=2
  Mux3 : Mux  Inputs=2
  Product : Product
  Product1 : Product
  Sin : Trigonometry
  Sum1 : Sum
  Sum2 : Sum  Inputs=+-
  R(theta)*p : Outport  VectorParamsAs1DForOutWhenUnconnected=off
  wires:
  p/1 -> Product/2, Product1/2
  Sum2/1 -> Mux3/2
  Sin/1 -> Product1/1
  theta/1 -> Cos/1, Sin/1
  Cos/1 -> Product/1
  Sum1/1 -> Mux3/1
  Mux3/1 -> R(theta)*p/1
  Product/1 -> Demux/1
  Product1/1 -> Demux1/1
  Demux/1 -> Sum1/1
  Demux1/2 -> Sum1/2
  Demux1/1 -> Sum2/2
  Demux/2 -> Sum2/1

== system Drone_BBall_Friendly/Drone 1 Dynamics/Quadcopter Plant/Rotational Dynamics/Wrap Angle ==
  raw : Inport
  Gain : Gain  Gain=2
  Mod : Math  Operator=mod  SignedPower=on  SaturateOnIntegerOverflow=on
  Pi : Constant  Value=pi  OutDataTypeStr=Inherit: Inherit via back propagation
  Sum3 : Sum  Inputs=|+-
  Sum4 : Sum  Inputs=|++
  wrap : Outport  VectorParamsAs1DForOutWhenUnconnected=off
  wires:
  Sum4/1 -> Mod/1
  Pi/1 -> Sum4/2, Sum3/2, Gain/1
  Sum3/1 -> wrap/1
  raw/1 -> Sum4/1
  Mod/1 -> Sum3/1
  Gain/1 -> Mod/2

== system Drone_BBall_Friendly/Drone 2 Dynamics/Hook Plant/Tether Dynamics/Rotation Matrix CW ==
  p : Inport
  theta : Inport  Port=2
  Cos : Trigonometry  Operator=cos
  Demux : Demux  Outputs=2
  Demux1 : Demux  Outputs=2
  Mux3 : Mux  Inputs=2
  Product : Product
  Product1 : Product
  Sin : Trigonometry
  Sum1 : Sum
  Sum2 : Sum  Inputs=+-
  R(theta)*p : Outport  VectorParamsAs1DForOutWhenUnconnected=off
  wires:
  p/1 -> Product/2, Product1/2
  Sum2/1 -> Mux3/2
  Sin/1 -> Product1/1
  theta/1 -> Cos/1, Sin/1
  Cos/1 -> Product/1
  Sum1/1 -> Mux3/1
  Mux3/1 -> R(theta)*p/1
  Product/1 -> Demux/1
  Product1/1 -> Demux1/1
  Demux/1 -> Sum1/1
  Demux1/2 -> Sum1/2
  Demux1/1 -> Sum2/2
  Demux/2 -> Sum2/1

== system Drone_BBall_Friendly/Drone 2 Dynamics/Quadcopter Plant/Rotational Dynamics/Wrap Angle ==
  raw : Inport
  Gain : Gain  Gain=2
  Mod : Math  Operator=mod  SignedPower=on  SaturateOnIntegerOverflow=on
  Pi : Constant  Value=pi  OutDataTypeStr=Inherit: Inherit via back propagation
  Sum3 : Sum  Inputs=|+-
  Sum4 : Sum  Inputs=|++
  wrap : Outport  VectorParamsAs1DForOutWhenUnconnected=off
  wires:
  Sum4/1 -> Mod/1
  Pi/1 -> Sum4/2, Sum3/2, Gain/1
  Sum3/1 -> wrap/1
  raw/1 -> Sum4/1
  Mod/1 -> Sum3/1
  Gain/1 -> Mod/2
